simulink model "DP2_simlink_refs"  (R2024b)
settings: Solver=FixedStepDiscrete  StartTime=0.0  StopTime=113800  FixedStep=1  RelTol=1e-3
undefined symbols (not defined in the file or in its folder): Ad, Bd, Cd, Dd, Pss, R_inv_pss
settings Model: Creator=zalak  LastModifiedBy=zalak

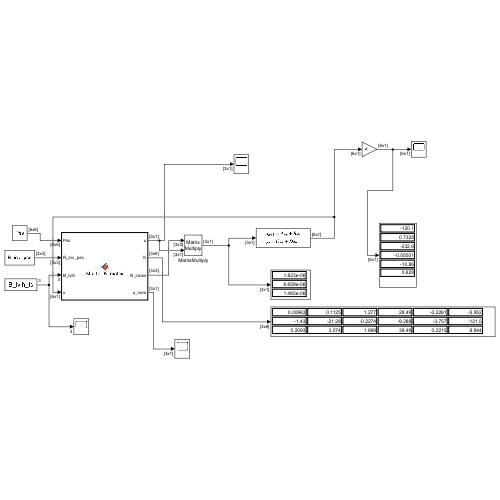
[thumbnail: Simulink's stored preview of the top-level diagram]
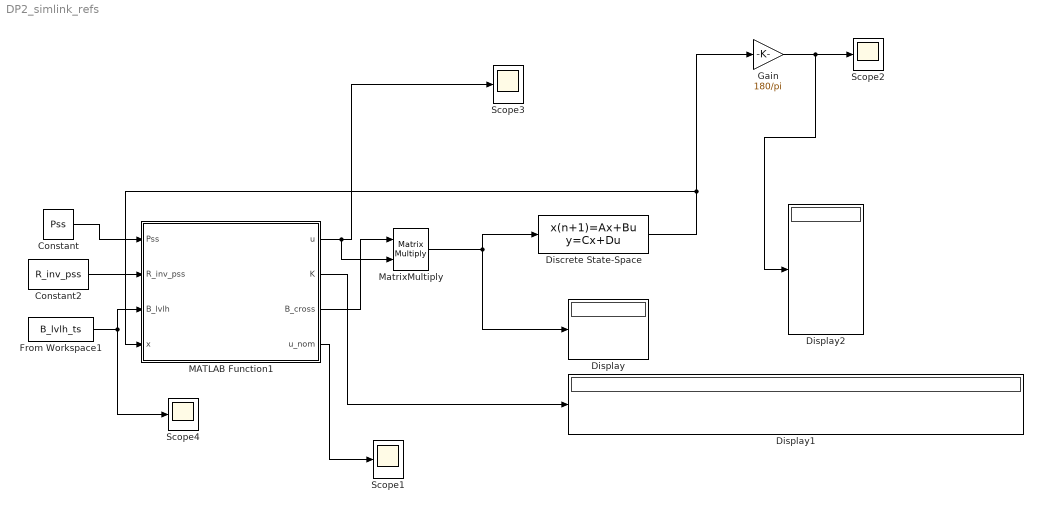
== system DP2_simlink_refs ==
  Constant : Constant  Value=Pss
  Constant2 : Constant  Value=R_inv_pss
  Discrete State-Space : DiscreteStateSpace  A=Ad  B=Bd  C=Cd  D=Dd  InitialCondition=[0.1*pi/180, 0, 0.1*pi/180, 0, 0.1*pi/180, 0]
  Display : Display
  Display1 : Display
  Display2 : Display
  From Workspace1 : FromWorkspace  VariableName=B_lvlh_ts  SampleTime=1
  Gain : Gain  Gain=180/pi
  MATLAB Function1 : MATLAB Function  TreatAsAtomicUnit=on
  MatrixMultiply : Product  Multiplication=Matrix(*)
  Scope{1..4} (4 alike) : Scope
  wires:
  Discrete State-Space/1 -> Gain/1, MATLAB Function1/4(x)
  Gain/1 -> Display2/1, Scope2/1
  From Workspace1/1 -> MATLAB Function1/3(B_lvlh), Scope4/1
  Constant/1 -> MATLAB Function1/1(Pss)
  Constant2/1 -> MATLAB Function1/2(R_inv_pss)
  MatrixMultiply/1 -> Display/1, Discrete State-Space/1
  MATLAB Function1/2(K) -> Display1/1
  MATLAB Function1/1(u) -> Scope3/1, MatrixMultiply/2
  MATLAB Function1/3(B_cross) -> MatrixMultiply/1
  MATLAB Function1/4(u_nom) -> Scope1/1

== matlab function DP2_simlink_refs/MATLAB Function1 ==
  data: Pss input; R_inv_pss input; B_lvlh input; x input; u output; K output; B_cross output; u_nom output
function [u, K, B_cross, u_nom] = lvlh_to_K_matrix(Pss, R_inv_pss, B_lvlh, x)
% Inputs -
%   Pss       (6×6)  constant periodic steady-state Riccati — from workspace
%   R_inv_pss (3×3)  must match R used to compute Pss — from workspace
%   B_lvlh    (3×1)  magnetic field in LVLH frame [T]
%   x         (6×1)  attitude error state

Ix = 0.00333;  Iy = 0.01020;  Iz = 0.01020;
m_max  = 0.166;    % A·m² — must match m_max_pss in setup script
alpha0 = 2.14;      % tuning scalar — start at 1, increase carefully
dt = 1;

%% LVLH → body rotation
phi = x(1);  theta = x(3);  psi = x(5);

Rx = [1,         0,          0;
      0,  cos(phi),  sin(phi);
      0, -sin(phi),  cos(phi)];
Ry = [cos(theta),  0, -sin(theta);
      0,           1,           0;
      sin(theta),  0,  cos(theta)];
Rz = [cos(psi),  sin(psi),  0;
     -sin(psi),  cos(psi),  0;
      0,         0,         1];

%% Constant B sanity check — comment out both lines below to use real B
%B_mean = 38.27e-6;
%B_body = [B_mean; B_mean; B_mean] / sqrt(3);   % unit direction, correct magnitude
B_body = Rz * Ry * Rx * B_lvlh(:);           % real B — uncomment when ready

Bx = B_body(1);  By = B_body(2);  Bz = B_body(3);

B_cross = [  0,   Bz,  -By;
            -Bz,   0,   Bx;
             By,  -Bx,   0];

B_tv = zeros(6,3);
B_tv(2,:) = B_cross(1,:) / Ix;
B_tv(4,:) = B_cross(2,:) / Iy;
B_tv(6,:) = B_cross(3,:) / Iz;

%% Gain — Pss constant, B_tv varies (or constant in this test)
K     = - alpha0 * R_inv_pss * (B_tv' * Pss);   % (3×6)
u_nom = K * x;                                % (3×1) [A·m²]

% Proportional saturation — Psiaki eq (2b)/(2c)
beta = max(abs(u_nom) / m_max);
if beta <= 1
    u = u_nom;
else
    u = u_nom / beta;   % scale all axes together, preserves direction
end

end
